simulink model "ikSolver"  (R2022a)
settings: Solver=VariableStepAuto  StartTime=0.0  StopTime=0  RelTol=1e-3
undefined symbols (not defined in the file or in its folder): Levenberg, Marquardt
libraries: robotcorelib x1, robotmaniplib x1
settings Model: Creator=The MathWorks, Inc.  LastModifiedBy=26794
settings SolverCC: AlgebraicLoopSolver=TrustRegion
settings DataIOCC: ReturnWorkspaceOutputs=off
settings DebuggingCC: UnconnectedInputMsg=warning  UnconnectedOutputMsg=warning  UnconnectedLineMsg=warning  SFMachineParentedDataDiag=warning  ArithmeticOperatorsInVariantConditions=warning
settings SFSimCC: SimUseLocalCustomCode=off  CustomCodeUndefinedFunction=UseInterfaceOnly
settings RTWCC: RTWUseLocalCustomCode=off

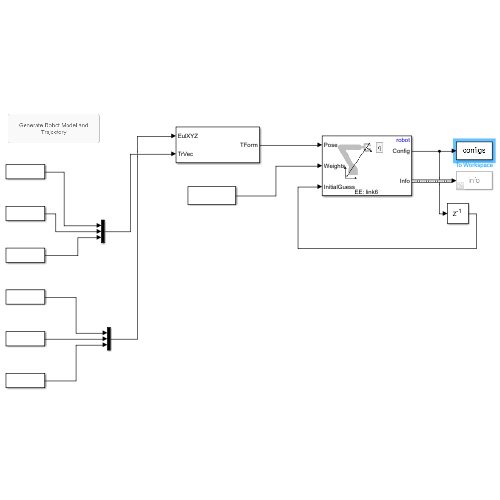
[thumbnail: Simulink's stored preview of the top-level diagram]
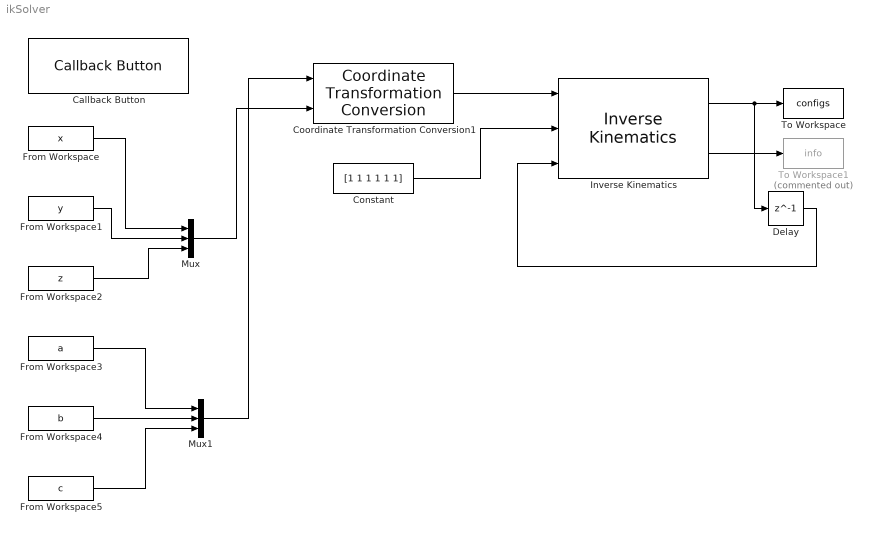
== system ikSolver ==
  Callback Button : CallbackButton  ButtonText=Generate Robot Model and Trajectory
      settings: ClickFcn=|
      | robot = importrobot('iiwa14.urdf');
      | robot.DataFormat = 'column';
      | x = 0.5*zeros(1,4)+0.25;
      | y = 0.25*[-1 -1 1 1];
      | z = 0.25*[-1 1 -1 1] + 0.75;
  Constant : Constant  Value=[1 1 1 1 1 1]
  Coordinate Transformation Conversion1 : robotcorelib/Coordinate Transformation Conversion  InputRepresentation=Euler Angles  InputEulerSequence=XYZ  ShowTrVecInputPort=on  OutputRepresentation=Homogeneous Transformation  OutputEulerSequence=ZYX  ShowTrVecOutputPort=on  SimulateUsing=Interpreted execution
      settings: SourceProductBaseCode=RO,NV,RR,UV
  Delay : Delay  DelayLength=1  InitialCondition=zeros(6,1)
  From Workspace : FromWorkspace  VariableName=x  OutDataTypeStr=double
  From Workspace1 : FromWorkspace  VariableName=y  OutDataTypeStr=double
  From Workspace2 : FromWorkspace  VariableName=z  OutDataTypeStr=double
  From Workspace3 : FromWorkspace  VariableName=a  OutDataTypeStr=double
  From Workspace4 : FromWorkspace  VariableName=b  OutDataTypeStr=double
  From Workspace5 : FromWorkspace  VariableName=c  OutDataTypeStr=double
  Inverse Kinematics : robotmaniplib/Inverse Kinematics  RigidBodyTree=robot  EndEffector=link6  ShowInfo=on  SolverName=Levenberg-Marquardt  EnforceJointLimits=on  MaxIterations=1500  MaxTime=10  GradientTolerance=1e-7  SolutionTolerance=1e-6  StepTolerance=1e-14  ErrorChangeTolerance=1e-12  UseErrorDamping=on  DampingBias=0.0025  SimulateUsing=Interpreted execution
  Mux : Mux  Inputs=3
  Mux1 : Mux  Inputs=3
  To Workspace : ToWorkspace  VariableName=configs  SaveFormat=Timeseries  SampleTime=0.01
  To Workspace1 : ToWorkspace  Commented=on  VariableName=info  SaveFormat=Timeseries  SampleTime=-1
  wires:
  From Workspace/1 -> Mux/1
  From Workspace1/1 -> Mux/2
  From Workspace2/1 -> Mux/3
  Constant/1 -> Inverse Kinematics/2
  Inverse Kinematics/1 -> Delay/1, To Workspace/1
  Inverse Kinematics/2 -> To Workspace1/1
  Delay/1 -> Inverse Kinematics/3
  From Workspace4/1 -> Mux1/2
  From Workspace3/1 -> Mux1/1
  From Workspace5/1 -> Mux1/3
  Mux1/1 -> Coordinate Transformation Conversion1/1
  Mux/1 -> Coordinate Transformation Conversion1/2
  Coordinate Transformation Conversion1/1 -> Inverse Kinematics/1
